simulink model "ecupolinominales"  (R2013a)
settings: Solver=ode45  StartTime=0.0  StopTime=20  RelTol=1e-3
settings Model: Creator=Daniel  LastModifiedBy=Daniel

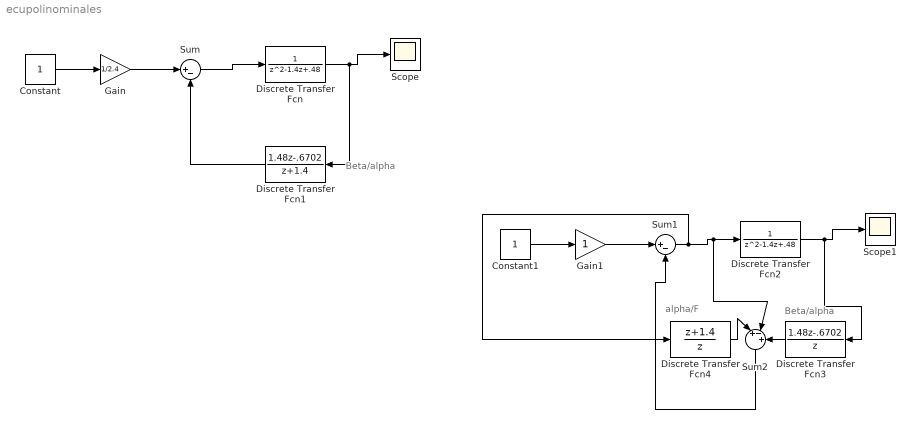
== system ecupolinominales ==
  note: Beta/alpha
  note: alpha/F
  note: Beta/alpha
  Constant : Constant
  Constant1 : Constant
  Discrete Transfer Fcn : DiscreteTransferFcn  Denominator="[1  -1.4 .48]"  SampleTime=1
  Discrete Transfer Fcn1 : DiscreteTransferFcn  Numerator=[1.48 -.6702]  Denominator=[1 1.4]
  Discrete Transfer Fcn2 : DiscreteTransferFcn  Denominator="[1  -1.4 .48]"  SampleTime=1
  Discrete Transfer Fcn3 : DiscreteTransferFcn  Numerator=[1.48 -.6702]  Denominator=[1 0]
  Discrete Transfer Fcn4 : DiscreteTransferFcn  Numerator=[1 1.4]  Denominator=[1 0]
  Gain : Gain  Gain=1/2.4
  Gain1 : Gain
  Scope : Scope
  Scope1 : Scope
  Sum : Sum  Inputs=|+-
  Sum1 : Sum  Inputs=|+-
  Sum2 : Sum  Inputs=|+-+
  wires:
  Gain/1 -> Sum/1
  Constant/1 -> Gain/1
  Sum/1 -> Discrete Transfer Fcn/1
  Discrete Transfer Fcn1/1 -> Sum/2
  Discrete Transfer Fcn/1 -> Discrete Transfer Fcn1/1, Scope/1
  Gain1/1 -> Sum1/1
  Constant1/1 -> Gain1/1
  Discrete Transfer Fcn2/1 -> Scope1/1, Discrete Transfer Fcn3/1
  Sum2/1 -> Sum1/2
  Discrete Transfer Fcn4/1 -> Sum2/1
  Sum1/1 -> Discrete Transfer Fcn4/1, Sum2/2, Discrete Transfer Fcn2/1
  Discrete Transfer Fcn3/1 -> Sum2/3
